simulink model "RRR_MPC_Nonlinear"  (R2024b)
settings: Solver=ode4  StartTime=0.0  StopTime=10.0  FixedStep=0.02  RelTol=1e-3
values from neighbouring files (symbols this model uses):
  q_star = [0; pi/4; -pi/6]    [compare.m]    (also in lin.m = [0; pi/4;-pi/6]; rrr_custom_mpc_block.m; rrr_linearmpc_block.m; rrr_mpc_relin.m = x_star(1:3))
  u_star = -robot.gravload(q_star')'    [compare.m]    (also in lin.m = G_star; rrr_custom_mpc_block.m = Gfun(q_star); rrr_linearmpc_block.m = Gfun(q_star); setup_RRR_MPC.m = G_star)
  x_star = [0; pi/4; -pi/6; 0; 0; 0]    [rrr_mpc_relin.m]    (also in setup_RRR_MPC.m = [q_star; zeros(3,1)])
libraries: mpclib x1
settings Model: Creator=Manuela  LastModifiedBy=Manuela

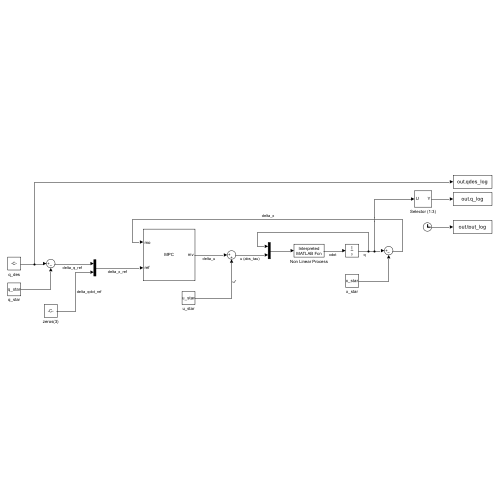
[thumbnail: Simulink's stored preview of the top-level diagram]
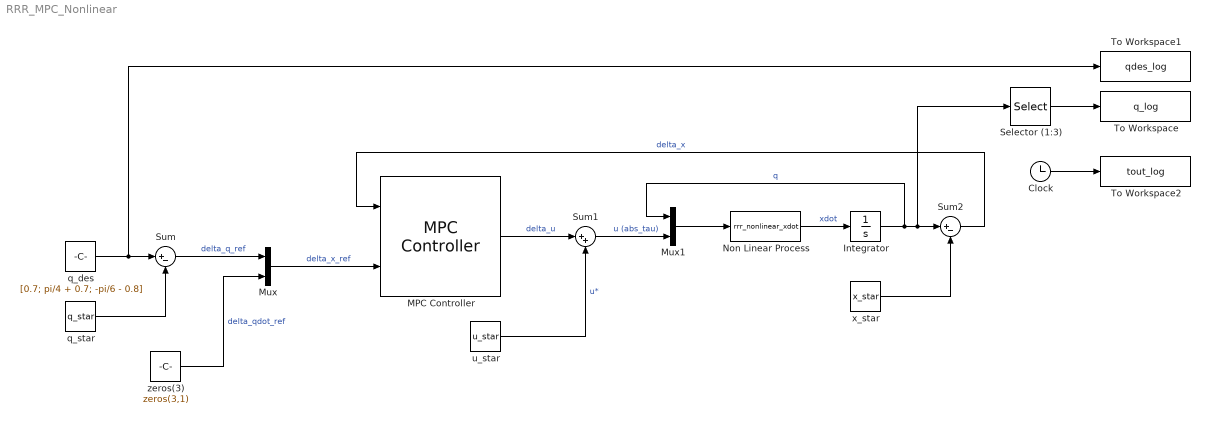
== system RRR_MPC_Nonlinear ==
  Clock : Clock
  Integrator : Integrator  InitialCondition=x_star
  MPC Controller : mpclib/MPC Controller  SCDEnableBlockLinearizationSpecification=on  mpcobj=mpcobj  is_multiple=0  enable_value=0  return_u0=off  updateMPCinCallerWorkspace=on  md_inport=off  mv_inport=off  uref_inport=off  return_cost=off  return_mvseq=off  return_qpstatus=off  return_xseq=off  return_state=off  return_ovseq=off  state_inport=off  umin_inport=off  umax_inport=off  ymin_inport=off  ymax_inport=off  cc_inport=off  ywt_inport=off  uwt_inport=off  duwt_inport=off  rhoeps_inport=off  pm_inport=off  MaximumP=10  HorizonChoice=FixedHorizon  n_ts=0.02  n_p=30  n_mv=3  n_md=0  n_ud=0  n_mo=6  n_uo=0  BlockDataType=double  SampleTimeInherited=off  switch_inport=off
  Mux : Mux  Inputs=2
  Mux1 : Mux  Inputs=2
  Non Linear Process : MATLABFcn  MATLABFcn=rrr_nonlinear_xdot  OutputDimensions=6
  Selector (1:3) : Selector  InputPortWidth=6  IndexOptions=Index vector (dialog)  Indices=[1 2 3]  OutputSizes=1
  Sum : Sum  Inputs=|+-
  Sum1 : Sum  Inputs=|++
  Sum2 : Sum  Inputs=|+-
  To Workspace : ToWorkspace  VariableName=q_log  SampleTime=-1
  To Workspace1 : ToWorkspace  VariableName=qdes_log  SampleTime=0.02
  To Workspace2 : ToWorkspace  VariableName=tout_log  SampleTime=-1
  q_des : Constant  Tag=q_des  Description=q_des  Value=[0.7; pi/4 + 0.7; -pi/6 - 0.8]  SampleTime=0.02
  q_star : Constant  Value=q_star
  u_star : Constant  Value=u_star
  x_star : Constant  Value=x_star
  zeros(3) : Constant  Value=zeros(3,1)
  wires:
  q_des/1 -> To Workspace1/1, Sum/1
  q_star/1 -> Sum/2
  Sum/1 -> Mux/1  "delta_q_ref"
  zeros(3)/1 -> Mux/2  "delta_qdot_ref"
  Mux/1 -> MPC Controller/2  "delta_x_ref"
  MPC Controller/1 -> Sum1/1  "delta_u"
  u_star/1 -> Sum1/2  "u*"
  Non Linear Process/1 -> Integrator/1  "xdot"
  x_star/1 -> Sum2/2
  Integrator/1 -> Selector (1:3)/1, Sum2/1, Mux1/1  "q"
  Sum1/1 -> Mux1/2  "u (abs_tau)"
  Mux1/1 -> Non Linear Process/1
  Sum2/1 -> MPC Controller/1  "delta_x"
  Selector (1:3)/1 -> To Workspace/1
  Clock/1 -> To Workspace2/1
